simulink model "IQRD_RLS_model_top"  (R2020b)
settings: Solver=VariableStepAuto  StartTime=0.0  StopTime=10.0  RelTol=1e-3
libraries: dspsrcs4 x3, simulink x2
settings Model: Creator=jgentile  LastModifiedBy=johngentile

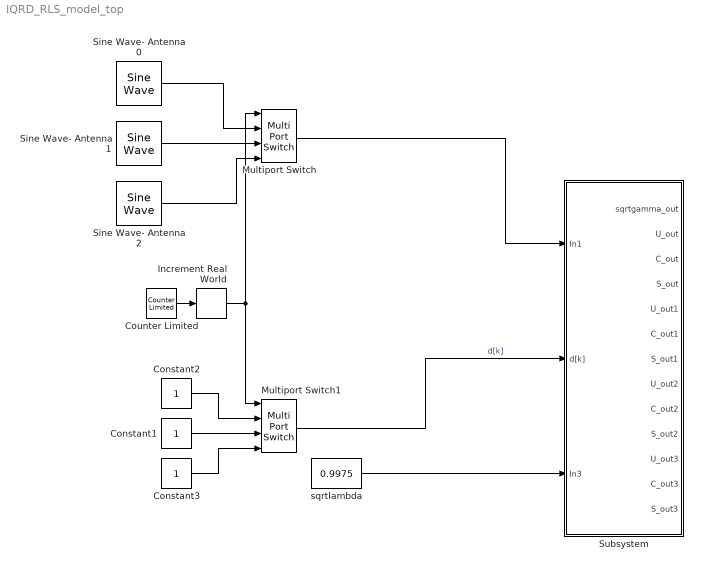
== system IQRD_RLS_model_top ==
  Constant1 : Constant
  Constant2 : Constant
  Constant3 : Constant
  Counter Limited : simulink/Sources/Counter Limited  uplimit=2  tsamp=-1
  Increment Real World : simulink/Additional Math & Discrete/Additional Math: Increment - Decrement/Increment Real World
      settings: SourceProductBaseCode=SL
  Multiport Switch : MultiPortSwitch
  Multiport Switch1 : MultiPortSwitch
  Sine Wave- Antenna 0 : dspsrcs4/Sine Wave  Amplitude=1  Frequency=100  Phase=0  SampleMode=Discrete  OutComplex=Complex  CompMethod=Trigonometric fcn  TableSize=Speed  SampleTime=1/1000  SamplesPerFrame=1  ResetState=Restart at time zero  OutputFrames=off  dataType=double  wordLen=16  udDataType=sfix(16)  fracBitsMode=Best precision  numFracBits=15  OutDataTypeStr=double  LastOutDataTypeStr=double
  Sine Wave- Antenna 1 : dspsrcs4/Sine Wave  Amplitude=1  Frequency=100  Phase=0  SampleMode=Discrete  OutComplex=Complex  CompMethod=Trigonometric fcn  TableSize=Speed  SampleTime=1/1000  SamplesPerFrame=1  ResetState=Restart at time zero  OutputFrames=off  dataType=double  wordLen=16  udDataType=sfix(16)  fracBitsMode=Best precision  numFracBits=15  OutDataTypeStr=double  LastOutDataTypeStr=double
  Sine Wave- Antenna 2 : dspsrcs4/Sine Wave  Amplitude=1  Frequency=100  Phase=0  SampleMode=Discrete  OutComplex=Complex  CompMethod=Trigonometric fcn  TableSize=Speed  SampleTime=1/1000  SamplesPerFrame=1  ResetState=Restart at time zero  OutputFrames=off  dataType=double  wordLen=16  udDataType=sfix(16)  fracBitsMode=Best precision  numFracBits=15  OutDataTypeStr=double  LastOutDataTypeStr=double
  Subsystem : Subsystem
  sqrtlambda : Constant  Value=0.9975
  wires:
  Sine Wave- Antenna 0/1 -> Multiport Switch/2
  Sine Wave- Antenna 1/1 -> Multiport Switch/3
  Sine Wave- Antenna 2/1 -> Multiport Switch/4
  Constant1/1 -> Multiport Switch1/3
  Constant2/1 -> Multiport Switch1/2
  Constant3/1 -> Multiport Switch1/4
  Counter Limited/1 -> Increment Real World/1
  Increment Real World/1 -> Multiport Switch1/1, Multiport Switch/1
  Multiport Switch/1 -> Subsystem/1(In1)
  Multiport Switch1/1 -> Subsystem/2(d[k])  "d[k]"
  sqrtlambda/1 -> Subsystem/3(In3)

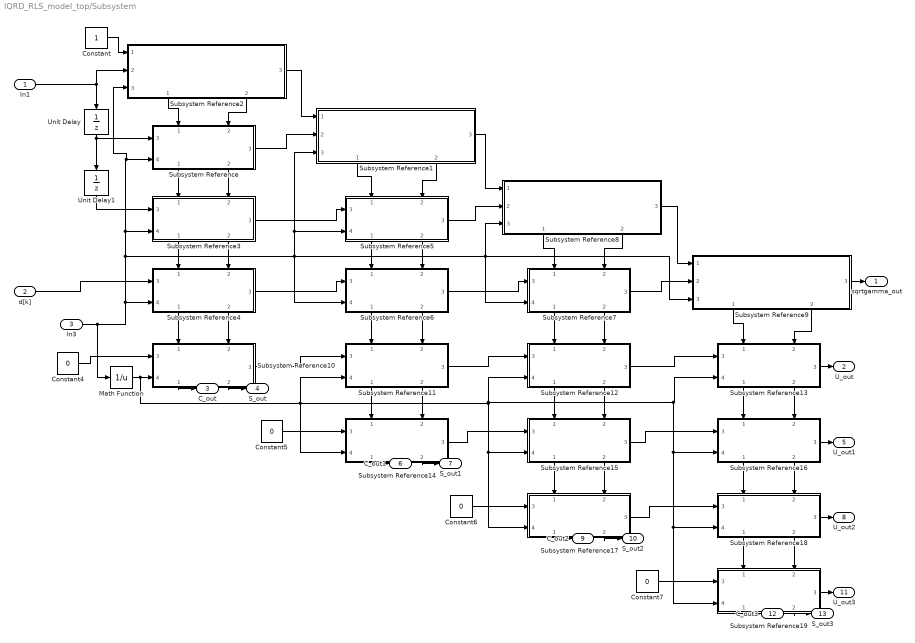
== system IQRD_RLS_model_top/Subsystem ==
  In1 : Inport
  d[k] : Inport  Port=2
  In3 : Inport  Port=3
  Constant : Constant
  Constant{4..7} (4 alike) : Constant  Value=0
  Math Function : Math  Operator=reciprocal  SaturateOnIntegerOverflow=on
  Subsystem Reference{,3..7,10..19} (16 alike) : Subsystem  ReferencedSubsystem=internal_cell_givens
      settings: PortSchema="{\"entries\":[{\"content\":{\"sides\":[{\"content\":{\"connectorIds\":[\"In3\",\"In4\"]},\"type\":\"ConnectorPlacement.EquallySpacedRectSide\",\"uuid\":\"0239e4e7-44b6-4143-a587-38d4cded4ca6\"},{\"content\":{\"connectorIds\":[\"Out3\"],\"side\":\"RIGHT\"},\"type\":\"ConnectorPlacement.EquallySpacedRectSide\",\"uuid\":\"ea23c866-1a25-41e9-a0f2-3862af1c86e1\"},{\"content\":{\"connectorIds\":[\"In1\",\"In2\"],\"side\":\"TOP\"},\"type\":\"ConnectorPlacement.EquallySpacedRectSide\",\"uuid\":\"8a8bb13e-2e16-40e7-9ca3-19d820578314\"},{\"content\":{\"connectorIds\":[\"Out1\",\"Out2\"],\"side\":\"BOTTOM\"},\"type\":\"ConnectorPlacement.EquallySpacedRectSide\",\"uuid\":\"1be66ea9-adc8-4a43-a798-b14d6fcab7cd\"},{\"content\":{\"connectorIds\":[],\"side\":\"HIDDEN\"},\"type\":\"ConnectorPlacement.EquallySpacedRectSide\",\"uuid\":\"0fecdaf4-55de-420b-b554-931c979049af\"}]},\"type\":\"ConnectorPlacement.EquallySpacedConnector\",\"uuid\":\"70182f79-db57-400d-a53f-39946a20555a\"}],\"packageUris\":[\"http://schema.mathworks.com/mf0/Connector/R2020b\"],\"version\":\"1.0\"}"
  Subsystem Reference{1..2,8..9} (4 alike) : Subsystem  ReferencedSubsystem=boundary_cell_givens
      settings: PortSchema="{\"entries\":[{\"content\":{\"sides\":[{\"content\":{\"connectorIds\":[\"In1\",\"In2\",\"In3\"]},\"type\":\"ConnectorPlacement.EquallySpacedRectSide\",\"uuid\":\"11c023aa-376d-416d-bfcd-8d7843f2be22\"},{\"content\":{\"connectorIds\":[\"Out3\"],\"side\":\"RIGHT\"},\"type\":\"ConnectorPlacement.EquallySpacedRectSide\",\"uuid\":\"1a04016b-daba-4444-ad99-d7273a1feb5b\"},{\"content\":{\"connectorIds\":[],\"side\":\"TOP\"},\"type\":\"ConnectorPlacement.EquallySpacedRectSide\",\"uuid\":\"dd6dcf65-02b5-4ffa-b5ff-7e58c587941b\"},{\"content\":{\"connectorIds\":[\"Out1\",\"Out2\"],\"side\":\"BOTTOM\"},\"type\":\"ConnectorPlacement.EquallySpacedRectSide\",\"uuid\":\"26ecda3d-5bd8-4d7b-b858-e25b16c314b4\"},{\"content\":{\"connectorIds\":[],\"side\":\"HIDDEN\"},\"type\":\"ConnectorPlacement.EquallySpacedRectSide\",\"uuid\":\"bd7630cc-a9b8-4021-b6b5-0e32bd520d7d\"}]},\"type\":\"ConnectorPlacement.EquallySpacedConnector\",\"uuid\":\"7bb81265-b299-46b6-8c47-6bc2be69935c\"}],\"packageUris\":[\"http://schema.mathworks.com/mf0/Connector/R2020b\"],\"version\":\"1.0\"}"
  Unit Delay : UnitDelay  SampleTime=-1  HasFrameUpgradeWarning=on
  Unit Delay1 : UnitDelay  SampleTime=-1  HasFrameUpgradeWarning=on
  sqrtgamma_out : Outport
  U_out : Outport  Port=2
  C_out : Outport  Port=3
  S_out : Outport  Port=4
  U_out1 : Outport  Port=5
  C_out1 : Outport  Port=6
  S_out1 : Outport  Port=7
  U_out2 : Outport  Port=8
  C_out2 : Outport  Port=9
  S_out2 : Outport  Port=10
  U_out3 : Outport  Port=11
  C_out3 : Outport  Port=12
  S_out3 : Outport  Port=13
  wires:
  Subsystem Reference10/2 -> S_out/1
  Subsystem Reference18/3 -> U_out2/1
  Subsystem Reference19/1 -> C_out3/1
  Subsystem Reference15/3 -> Subsystem Reference16/3
  Subsystem Reference18/1 -> Subsystem Reference19/1
  Subsystem Reference12/3 -> Subsystem Reference13/3
  Subsystem Reference11/3 -> Subsystem Reference12/3
  Subsystem Reference16/2 -> Subsystem Reference18/2
  Subsystem Reference2/1 -> Subsystem Reference/1
  Subsystem Reference15/1 -> Subsystem Reference17/1
  Subsystem Reference13/2 -> Subsystem Reference16/2
  Subsystem Reference7/2 -> Subsystem Reference12/2
  Subsystem Reference16/3 -> U_out1/1
  Subsystem Reference12/2 -> Subsystem Reference15/2
  Constant6/1 -> Subsystem Reference17/3
  Subsystem Reference4/1 -> Subsystem Reference10/1
  Subsystem Reference1/1 -> Subsystem Reference5/1
  Subsystem Reference6/2 -> Subsystem Reference11/2
  Subsystem Reference3/3 -> Subsystem Reference5/3
  Subsystem Reference11/1 -> Subsystem Reference14/1
  Subsystem Reference11/2 -> Subsystem Reference14/2
  Subsystem Reference19/3 -> U_out3/1
  Subsystem Reference/3 -> Subsystem Reference1/2
  Subsystem Reference4/3 -> Subsystem Reference6/3
  Subsystem Reference17/1 -> C_out2/1
  Subsystem Reference6/3 -> Subsystem Reference7/3
  In1/1 -> Unit Delay/1, Subsystem Reference2/2
  Subsystem Reference5/3 -> Subsystem Reference8/2
  Subsystem Reference19/2 -> S_out3/1
  Subsystem Reference12/1 -> Subsystem Reference15/1
  Subsystem Reference14/1 -> C_out1/1
  Subsystem Reference9/3 -> sqrtgamma_out/1
  Subsystem Reference3/2 -> Subsystem Reference4/2
  Subsystem Reference2/3 -> Subsystem Reference1/1
  Subsystem Reference6/1 -> Subsystem Reference11/1
  Constant7/1 -> Subsystem Reference19/3
  Subsystem Reference18/2 -> Subsystem Reference19/2
  Subsystem Reference14/3 -> Subsystem Reference15/3
  d[k]/1 -> Subsystem Reference4/3
  Subsystem Reference/1 -> Subsystem Reference3/1
  Subsystem Reference13/3 -> U_out/1
  Subsystem Reference14/2 -> S_out1/1
  Constant5/1 -> Subsystem Reference14/3
  Subsystem Reference7/3 -> Subsystem Reference9/2
  Subsystem Reference3/1 -> Subsystem Reference4/1
  Subsystem Reference/2 -> Subsystem Reference3/2
  Constant/1 -> Subsystem Reference2/1
  Subsystem Reference17/2 -> S_out2/1
  Subsystem Reference7/1 -> Subsystem Reference12/1
  Constant4/1 -> Subsystem Reference10/3
  In3/1 -> Math Function/1, Subsystem Reference3/4, Subsystem Reference2/3, Subsystem Reference/4, Subsystem Reference8/3, Subsystem Reference9/3, Subsystem Reference7/4, Subsystem Reference6/4, Subsystem Reference5/4, Subsystem Reference1/3, Subsystem Reference4/4
  Subsystem Reference10/3 -> Subsystem Reference11/3
  Unit Delay1/1 -> Subsystem Reference3/3
  Subsystem Reference9/2 -> Subsystem Reference13/2
  Subsystem Reference10/1 -> C_out/1
  Subsystem Reference1/3 -> Subsystem Reference8/1
  Subsystem Reference5/2 -> Subsystem Reference6/2
  Subsystem Reference9/1 -> Subsystem Reference13/1
  Subsystem Reference5/1 -> Subsystem Reference6/1
  Subsystem Reference2/2 -> Subsystem Reference/2
  Subsystem Reference16/1 -> Subsystem Reference18/1
  Subsystem Reference8/3 -> Subsystem Reference9/1
  Subsystem Reference4/2 -> Subsystem Reference10/2
  Math Function/1 -> Subsystem Reference14/4, Subsystem Reference19/4, Subsystem Reference18/4, Subsystem Reference16/4, Subsystem Reference13/4, Subsystem Reference12/4, Subsystem Reference17/4, Subsystem Reference15/4, Subsystem Reference11/4, Subsystem Reference10/4
  Subsystem Reference15/2 -> Subsystem Reference17/2
  Unit Delay/1 -> Unit Delay1/1, Subsystem Reference/3
  Subsystem Reference8/2 -> Subsystem Reference7/2
  Subsystem Reference1/2 -> Subsystem Reference5/2
  Subsystem Reference13/1 -> Subsystem Reference16/1
  Subsystem Reference17/3 -> Subsystem Reference18/3
  Subsystem Reference8/1 -> Subsystem Reference7/1
